simulink model "Q5_parity"  (R2021b)
settings: Solver=VariableStepAuto  StartTime=0.0  StopTime=10.0  RelTol=1e-3
undefined symbols (not defined in the file or in its folder): A_d, B_d, Hd_s, Hf_s, Hu_s, V_s, V_s_nd
settings Model: Creator=user  LastModifiedBy=user

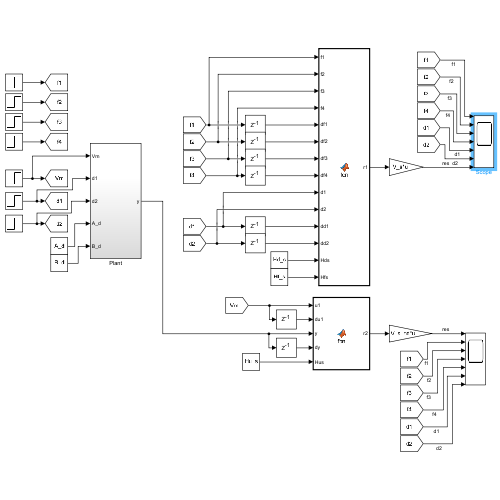
[thumbnail: Simulink's stored preview of the top-level diagram]
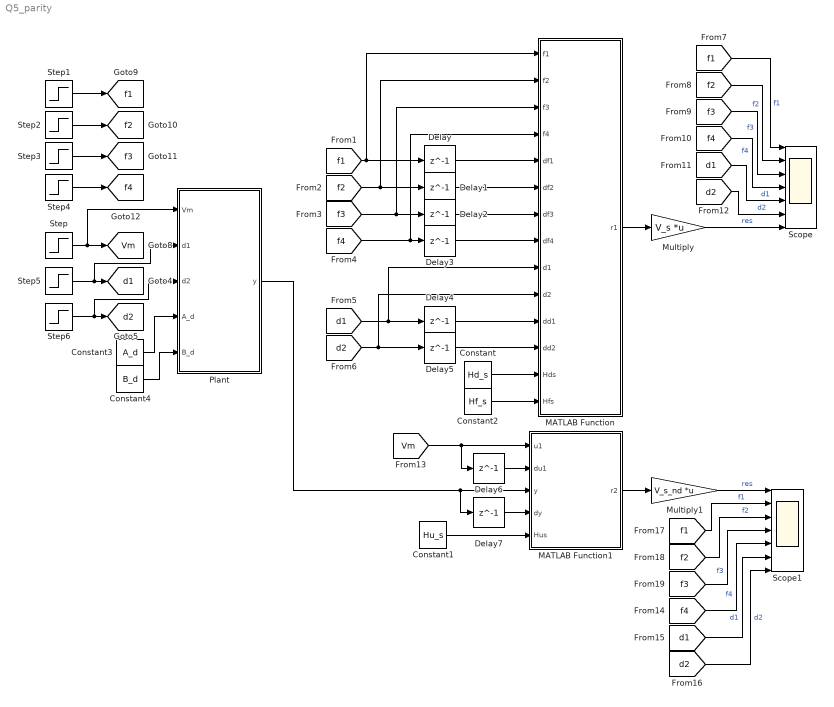
== system Q5_parity ==
  Constant : Constant  Value=Hd_s
  Constant1 : Constant  Value=Hu_s
  Constant2 : Constant  Value=Hf_s
  Constant3 : Constant  Value=A_d
  Constant4 : Constant  Value=B_d
  Delay{,1..7} (8 alike) : Delay  DelayLength=1  InitialCondition=0
  MATLAB Function : MATLAB Function  TreatAsAtomicUnit=on
  MATLAB Function1 : MATLAB Function  TreatAsAtomicUnit=on
  Multiply : Gain  Gain=V_s  Multiplication=Matrix(K*u)
  Multiply1 : Gain  Gain=V_s_nd  Multiplication=Matrix(K*u)
  Plant : Subsystem
  Scope : Scope  NumInputPorts=7
  Scope1 : Scope  NumInputPorts=7
  Step : Step  Time=2  Before=1  After=5  SampleTime=0
  Step1 : Step  After=2  SampleTime=0
  Step2 : Step  Time=2  After=2  SampleTime=0
  Step3 : Step  Time=3  After=2  SampleTime=0
  Step4 : Step  Time=4  After=3  SampleTime=0
  Step5 : Step  Time=2.5  After=0.1  SampleTime=0
  Step6 : Step  Time=4.5  After=0.2  SampleTime=0
  tag scope: Vm=global, d1=global, d2=global, f1=global, f2=global, f3=global, f4=global
  wires:
  Step4/1 -> [f4]
  Step/1 -> Plant/1(Vm), [Vm]
  Step1/1 -> [f1]
  Step3/1 -> [f3]
  Step2/1 -> [f2]
  [f1] -> MATLAB Function/1(f1), Delay/1
  [f2] -> MATLAB Function/2(f2), Delay1/1
  [f3] -> MATLAB Function/3(f3), Delay2/1
  [f4] -> MATLAB Function/4(f4), Delay3/1
  Step5/1 -> Plant/2(d1), [d1]
  Step6/1 -> Plant/3(d2), [d2]
  [d2] -> MATLAB Function/10(d2), Delay5/1
  [d1] -> MATLAB Function/9(d1), Delay4/1
  Delay/1 -> MATLAB Function/5(df1)
  Delay1/1 -> MATLAB Function/6(df2)
  Delay2/1 -> MATLAB Function/7(df3)
  Delay3/1 -> MATLAB Function/8(df4)
  Delay4/1 -> MATLAB Function/11(dd1)
  Delay5/1 -> MATLAB Function/12(dd2)
  Constant/1 -> MATLAB Function/13(Hds)
  Constant2/1 -> MATLAB Function/14(Hfs)
  Constant3/1 -> Plant/4(A_d)
  Constant4/1 -> Plant/5(B_d)
  MATLAB Function/1(r1) -> Multiply/1
  Multiply/1 -> Scope/7  "res"
  [f1] -> Scope/1  "f1"
  [f2] -> Scope/2  "f2"
  [f3] -> Scope/3  "f3"
  [f4] -> Scope/4  "f4"
  [d1] -> Scope/5  "d1"
  [d2] -> Scope/6  "d2"
  [Vm] -> Delay6/1, MATLAB Function1/1(u1)
  Delay6/1 -> MATLAB Function1/2(du1)
  Plant/1(y) -> Delay7/1, MATLAB Function1/3(y)
  Delay7/1 -> MATLAB Function1/4(dy)
  Constant1/1 -> MATLAB Function1/5(Hus)
  MATLAB Function1/1(r2) -> Multiply1/1
  Multiply1/1 -> Scope1/1  "res"
  [f4] -> Scope1/5  "f4"
  [f2] -> Scope1/3  "f2"
  [d2] -> Scope1/7  "d2"
  [f3] -> Scope1/4  "f3"
  [d1] -> Scope1/6  "d1"
  [f1] -> Scope1/2  "f1"

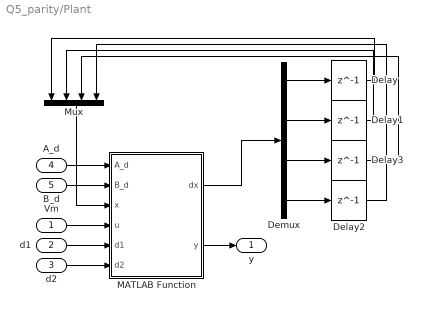
== system Q5_parity/Plant ==
  Vm : Inport
  d1 : Inport  Port=2
  d2 : Inport  Port=3
  A_d : Inport  Port=4
  B_d : Inport  Port=5
  Delay{,1..3} (4 alike) : Delay  DelayLength=1  InputProcessing=Columns as channels (frame based)
  Demux : Demux
  MATLAB Function : MATLAB Function  TreatAsAtomicUnit=on
  Mux : Mux
  y : Outport
  wires:
  Vm/1 -> MATLAB Function/4(u)
  Mux/1 -> MATLAB Function/3(x)
  Demux/1 -> Delay/1
  Demux/2 -> Delay1/1
  Demux/3 -> Delay3/1
  Demux/4 -> Delay2/1
  Delay/1 -> Mux/1
  Delay1/1 -> Mux/2
  Delay3/1 -> Mux/3
  Delay2/1 -> Mux/4
  d1/1 -> MATLAB Function/5(d1)
  d2/1 -> MATLAB Function/6(d2)
  B_d/1 -> MATLAB Function/2(B_d)
  A_d/1 -> MATLAB Function/1(A_d)
  MATLAB Function/2(y) -> y/1
  MATLAB Function/1(dx) -> Demux/1

== matlab function Q5_parity/MATLAB Function ==
  data: f1 input; r1 output; f2 input; f3 input; f4 input; df1 input; df2 input; df3 input; df4 input; d1 input; d2 input; dd1 input; dd2 input; Hds input; Hfs input
function r1 = fcn(f1,f2,f3,f4,df1,df2,df3,df4,d1,d2,dd1,dd2,Hds,Hfs)
d=[dd1;d1;dd2;d2];
f=[df1;f1;df2;f2;df3;f3;df4;f4];
r1 = (Hds*d + Hfs*f);

== matlab function Q5_parity/Plant/MATLAB Function ==
  data: dx output; A_d input; B_d input; x input; u input; d1 input; d2 input; y output
function [dx,y]  = plant(A_d,B_d,x,u,d1,d2)
dx = zeros(4,1);
A=A_d;
B = B_d;
C = eye(4);
E=[1 0;0 1;0 0;0 0];
temp = A*x;
temp2 = B*u;
temp3 = E*[d1;d2];
y=C*x;
%y = size(dx,1);
end

== matlab function Q5_parity/MATLAB Function1 ==
  data: u1 input; r2 output; du1 input; y input; dy input; Hus input
function r2 = fcn(u1,du1,y,dy,Hus)
y=[dy;y];
u=[du1;u1];
r2 = y-Hus*u;
